simulink model "UNIFIER_3DOFsim"  (R2023b)
settings: Solver=VariableStepAuto  StartTime=0  StopTime=t_sim  RelTol=1e-3
InitFcn:
  | UNIFIER_3DOFsim_init
values from neighbouring files (symbols this model uses):
  b = 20.11467    [UNIFIER_LOAD.m]    (also in UNIFIER_LOAD.mat; UNIFIER_LOAD_ROM.m; UNIFIER_LOAD_ROM.mat)
  c = 1.43676    [UNIFIER_LOAD.m]    (also in UNIFIER_LOAD.mat; UNIFIER_LOAD_ROM.m; UNIFIER_LOAD_ROM.mat)
  DEP_inc = -0.0872664625997    [UNIFIER_LOAD.mat]    (also in UNIFIER_ROMdyn.m = deg2rad(-5); UNIFIER_ROMdyn_script.m = deg2rad(-5); UNIFIER_ROMdyn_v2.m = deg2rad(-5); UNIFIER_ROMgen.m = 0.1)
  dp_DEP =     [UNIFIER_LOAD.mat]    (also in UNIFIER_LOAD_ROM.mat)
  dp_FUSE_FIN =     [UNIFIER_LOAD.mat]
  dp_HTU =     [UNIFIER_LOAD.mat]    (also in UNIFIER_LOAD_ROM.mat)
  dp_VTAIL =     [UNIFIER_LOAD.mat]
  dp_VTAIL_INDUCED =     [UNIFIER_LOAD.mat]
  dp_WING_root =     [UNIFIER_LOAD.mat]
  dp_WING_tip =     [UNIFIER_LOAD.mat]
  dumax = [2.09439510239 2.09439510239 2.09439510239 1.0471975512 2 4 2]    [UNIFIER_LOAD.mat]    (also in UNIFIER_LOAD_ROM.mat = [1.0471975512 1.0471975512 1.0471975512 0.174532925199 2 2 2)
  gr = 9.80665    [UNIFIER_LOAD.mat]    (also in UNIFIER_LOAD_ROM.mat)
  m = 7057    [UNIFIER_LOAD.m]    (also in UNIFIER_LOAD.mat; UNIFIER_LOAD_ROM.m; UNIFIER_LOAD_ROM.mat)
  n_prop = 12    [UNIFIER_LOAD.mat]    (also in UNIFIER_ROMdyn.m; UNIFIER_ROMdyn_script.m; UNIFIER_ROMdyn_v2.m)
  prop_d = 1.6    [UNIFIER_LOAD.mat]    (also in UNIFIER_ROMdyn.m; UNIFIER_ROMdyn_script.m; UNIFIER_ROMdyn_v2.m)
  ROMv1 = ROM    [UNIFIER_3DOFsim_init.m]    (also in UNIFIER_ROMgen_subset.m; UNIFIER_ROMgen_v2_subset.m; UNIFIER_ROMgen_v3_subset.m; UNIFIER_ROMgen_v4_subset.m)
  ROMv2 = ROM    [UNIFIER_3DOFsim_init.m]
  ROMv3 = ROM    [UNIFIER_3DOFsim_init.m]
  S = 29.98388    [UNIFIER_LOAD.m]    (also in UNIFIER_LOAD.mat; UNIFIER_LOAD_ROM.m; UNIFIER_LOAD_ROM.mat)
  U_trim = [ustar(3) ... (first row only)    [UNIFIER_3DOFsim_init.m]
  umax = inf    [UNIFIERLanding.m]    (also in UNIFIER_LOAD.mat = [0.436332312999 0.523598775598 0.523598775598 0.436332312999; UNIFIER_LOAD_ROM.mat = [0.436332312999 0.523598775598 0.349065850399 0.436332312999)
  umin = 0    [UNIFIERLanding.m]    (also in UNIFIER_LOAD.mat = [-0.436332312999 -0.523598775598 -0.523598775598 0 0 -1 -0.5; UNIFIER_LOAD_ROM.mat = [-0.436332312999 -0.523598775598 -0.0872664625997 0 0 -1 0])
  Va = sqrt(u^2+w^2)    [ROMcomp.m]    (also in UNIFIERLanding.m = sqrt(x(:,3).^2+x(:,4).^2); UNIFIERLanding_Dynamics_Internal.m = sqrt(X(:,3).^2+X(:,4).^2); UNIFIERLanding_Main.m = sqrt(solution.X(:,3).^2+solution.X(:,4).^2); UNIFIERLanding_trajopt.m = sqrt(solution.X(:,3).^2+solution.X(:,4).^2))
  vtail_nodes = [dp_VTAIL.Xs_LE;     dp_VTAIL.Ys_LE;     dp_VTAIL.Zs_LE]    [UNIFIER_LOAD.m]    (also in UNIFIER_LOAD.mat = [-16.4894695282 -2.83441376686 -2.73765826225 -16.1370849609)
  wing_nodes = [fliplr(dp_WING_tip.LE_Xs),fliplr(dp_WING_root.LE_Xs),dp_WING_root.LE_Xs,dp_WING_tip.LE_Xs;     fliplr(-dp_WING_tip.LE_Ys),fliplr(-dp_WING_root.LE_Ys),dp_WING_root.LE_Ys,dp_WING_tip.LE_Ys;     fliplr(dp_WING_tip.LE_Zs),fliplr(dp_WING_root.LE_Zs),dp_WING_root.LE_Zs,dp_WING_tip.LE_Zs]    [UNIFIER_LOAD.m]    (also in UNIFIER_LOAD.mat = [-7.70795631409 -9.67500019073 -0.98178178072 -7.66801691055)
  x0 = xstar(1)    [UNIFIERLanding.m]    (also in UNIFIER_3DOFsim_init.m; UNIFIER_dynamics.m = x; UNIFIER_trim.m = [Va_target/100; UNIFIER_trim1.m = [Va_target)
  xstar = [0;        0;        -ze_target;        zstar(1)*100;        0;        zstar(2)*100;        0;        zstar(3);        0;        0;        0;        0]    [UNIFIER_trim.m]    (also in UNIFIER_trim0_res.mat = [0 0 -500 55.1327882403 0 -0.446351795968 0 1.36591182427e-0; UNIFIER_trim1.m = [0;        0;        -ze_target;        zstar(1);        0; ; UNIFIER_trim1_res.mat = [0 0 -1219 72.7310470326 0 1.14230710452 0 0.0157060522827 0; UNIFIER_trimHFM.m = [0;        0;        -runconfig.ze;        zstar(1)*100;    )
  xyz_cg = [-8.09,0,-0.2]    [UNIFIER_LOAD.m]    (also in UNIFIER_LOAD.mat = [-8.09 0 -0.2]; UNIFIER_LOAD_ROM.m; UNIFIER_LOAD_ROM.mat = [-8.09 0 -0.2])
  xyz_cg_12 = [-8.09 0 -0.2 -8.09 0 -0.2 -8.09 0 -0.2 -8.09 0 -0.2 ... (36 elements, 3x12)]    [UNIFIER_LOAD.mat]    (also in UNIFIER_LOAD_ROM.mat)
  xyz_DEP = [ -6.9629998	-6.9210000	-6.8660002	-6.8099999	-6.7540002	-6.6999998	-6.6999998	-6.7540002	-6.8099999	-6.8660002	-6.9210000	-6.9629998 ... (first row only)    [UNIFIER_LOAD.m]    (also in UNIFIER_LOAD.mat = [-6.9629998 -10.05 -0.90899998 -6.921 -8.4499998 -0.792 -6.8; UNIFIER_LOAD_ROM.m; UNIFIER_LOAD_ROM.mat = [-6.9629998 -10.05 -0.90899998 -6.921 -8.4499998 -0.792 -6.8)
  z0 = x(1,2)    [UNIFIERLanding.m]    (also in UNIFIER_3DOFsim_init.m = xstar(3); UNIFIER_trim.m = zstar; UNIFIER_trim1.m = zstar; UNIFIER_trimHFM.m = zstar)
undefined symbols (not defined in the file or in its folder): solution
libraries: simulink_extras x17, sharedutil x5, slpidlib x4, aerolibtransform2 x4, dspindex x2, matrix_library x1, shared6dof x1, aerolibatmos2 x1, simulink x1
(part 4 of 4)

== system UNIFIER_3DOFsim/UNIFIER/Aerodynamics/HFM/Aero/WingForces/Right/WingRootForces/WingRootPreLookup ==
  flap_defl : Inport
  alpha : Inport  Port=2
  V_node : Inport  Port=3
  DEP_J : Inport  Port=4
  Constant8 : Constant  Value=0:4
  Prelookup : PreLookup  BreakpointsData=dp_WING_root.flap_defl  IndexSearchMethod=Linear search  BeginIndexSearchUsingPreviousIndexResult=on  UseLastBreakpoint=on
  Prelookup1 : PreLookup  BreakpointsData=dp_WING_root.alphas  IndexSearchMethod=Linear search  BeginIndexSearchUsingPreviousIndexResult=on  UseLastBreakpoint=on
  Prelookup2 : PreLookup  BreakpointsData=dp_WING_root.V  IndexSearchMethod=Linear search  BeginIndexSearchUsingPreviousIndexResult=on  UseLastBreakpoint=on
  Prelookup3 : PreLookup  BreakpointsData=dp_WING_root.DEP_J  IndexSearchMethod=Linear search  BeginIndexSearchUsingPreviousIndexResult=on  UseLastBreakpoint=on
  Out1 : Outport
  Out2 : Outport  Port=2
  Out3 : Outport  Port=3
  Out4 : Outport  Port=4
  Out6 : Outport  Port=5
  Out7 : Outport  Port=6
  Out8 : Outport  Port=7
  Out9 : Outport  Port=8
  Out5 : Outport  Port=9
  wires:
  Prelookup3/2 -> Out9/1
  Prelookup3/1 -> Out8/1
  Prelookup2/2 -> Out7/1
  Prelookup2/1 -> Out6/1
  DEP_J/1 -> Prelookup3/1
  V_node/1 -> Prelookup2/1
  flap_defl/1 -> Prelookup/1
  Prelookup1/1 -> Out3/1
  alpha/1 -> Prelookup1/1
  Prelookup/2 -> Out2/1
  Prelookup1/2 -> Out4/1
  Constant8/1 -> Out5/1
  Prelookup/1 -> Out1/1

== system UNIFIER_3DOFsim/UNIFIER/Aerodynamics/HFM/Aero/WingForces/Right/WingTipForces/WingRootPreLookup ==
  ail_defl : Inport
  alpha : Inport  Port=2
  V_node : Inport  Port=3
  DEP_J : Inport  Port=4
  Constant8 : Constant  Value=0:1
  Prelookup : PreLookup  BreakpointsData=dp_WING_tip.ail_defl  IndexSearchMethod=Linear search  BeginIndexSearchUsingPreviousIndexResult=on  UseLastBreakpoint=on
  Prelookup1 : PreLookup  BreakpointsData=dp_WING_tip.alphas  IndexSearchMethod=Linear search  BeginIndexSearchUsingPreviousIndexResult=on  UseLastBreakpoint=on
  Prelookup2 : PreLookup  BreakpointsData=dp_WING_tip.V  IndexSearchMethod=Linear search  BeginIndexSearchUsingPreviousIndexResult=on  UseLastBreakpoint=on
  Prelookup3 : PreLookup  BreakpointsData=dp_WING_tip.DEP_J  IndexSearchMethod=Linear search  BeginIndexSearchUsingPreviousIndexResult=on  UseLastBreakpoint=on
  Out1 : Outport
  Out2 : Outport  Port=2
  Out3 : Outport  Port=3
  Out4 : Outport  Port=4
  Out6 : Outport  Port=5
  Out7 : Outport  Port=6
  Out8 : Outport  Port=7
  Out9 : Outport  Port=8
  Out5 : Outport  Port=9
  wires:
  Prelookup3/2 -> Out9/1
  Prelookup3/1 -> Out8/1
  Prelookup2/2 -> Out7/1
  Prelookup2/1 -> Out6/1
  DEP_J/1 -> Prelookup3/1
  V_node/1 -> Prelookup2/1
  ail_defl/1 -> Prelookup/1
  Prelookup1/1 -> Out3/1
  alpha/1 -> Prelookup1/1
  Prelookup/2 -> Out2/1
  Prelookup1/2 -> Out4/1
  Constant8/1 -> Out5/1
  Prelookup/1 -> Out1/1
